simulink model "PIDPitch"  (R2012b)
settings: Solver=FixedStepDiscrete  StartTime=0.0  StopTime=9.96  FixedStep=Ts  RelTol=1e-3
values from neighbouring files (symbols this model uses):
  esc = esc+1    [bateria.m]
undefined symbols (not defined in the file or in its folder): DiscIntNeverNeededParam, Ts
libraries: simulink x2, slident x1
settings Model: Creator=TOSHIBA  LastModifiedBy=Carlos
settings ConfigurationSet: Description=SimMechanics 2G

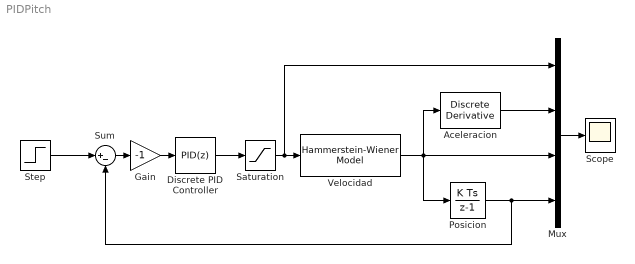
== system PIDPitch ==
  Aceleracion : simulink/Discrete/Discrete Derivative  gainval=1.0  ICPrevScaledInput=0.0  InputProcessing=Inherited  OutMin=[]  OutMax=[]  OutDataType=fixdt(1, 16)  OutScaling=2^-10  DoSatur=off
  Discrete PID Controller : simulink/Continuous/PID Controller  Controller=PID  TimeDomain=Discrete-time  SampleTime=Ts  IntegratorMethod=Forward Euler  FilterMethod=Forward Euler  Form=Parallel  P=0.7  I=0  D=0.5  N=15  InitialConditionSource=internal  InitialConditionForIntegrator=0  InitialConditionForFilter=0  ExternalReset=none  LimitOutput=off  UpperSaturationLimit=inf  LowerSaturationLimit=-inf  LinearizeAsGain=off  AntiWindupMode=none  Kb=1  TrackingMode=off  Kt=1  PParamMin=[]  PParamMax=[]  IParamMin=[]  IParamMax=[]  DParamMin=[]  DParamMax=[]  NParamMin=[]  NParamMax=[]  KbParamMin=[]  KbParamMax=[]  KtParamMin=[]  KtParamMax=[]  POutMin=[]  POutMax=[]  IOutMin=[]  IOutMax=[]  DOutMin=[]  DOutMax=[]  NOutMin=[]  NOutMax=[]  KbOutMin=[]  KbOutMax=[]  KtOutMin=[]  KtOutMax=[]  IntegratorOutMin=[]  IntegratorOutMax=[]  FilterOutMin=[]  FilterOutMax=[]  SumOutMin=[]  SumOutMax=[]  SumI1OutMin=[]  SumI1OutMax=[]  SumI2OutMin=[]  SumI2OutMax=[]  SumI3OutMin=[]  SumI3OutMax=[]  SumDOutMin=[]  SumDOutMax=[]  SaturationOutMin=[]  SaturationOutMax=[]  IntegratorContinuousStateAttributes=''  IntegratorStateMustResolveToSignalObject=off  IntegratorRTWStateStorageClass=Auto  FilterContinuousStateAttributes=''  FilterStateMustResolveToSignalObject=off  FilterRTWStateStorageClass=Auto
  Gain : Gain  Gain=-1  SampleTime=Ts
  Mux : Mux
  Posicion : DiscreteIntegrator  SampleTime=Ts  ICPrevOutput=DiscIntNeverNeededParam  ICPrevScaledInput=DiscIntNeverNeededParam
  Saturation : Saturate  UpperLimit=1  LowerLimit=-1  SampleTime=Ts
  Scope : Scope
      settings: SaveName=scdatavx  SampleInput=on  SampleTime=Ts
  Step : Step  After=esc  SampleTime=Ts
  Sum : Sum  Inputs=|+-  SampleTime=Ts
  Velocidad : slident/Hammerstein-Wiener Model  sys=vx123_nlhw113_pic2  IC=Zero  X0i=0
  wires:
  Velocidad/1 -> Aceleracion/1, Mux/3, Posicion/1
  Step/1 -> Sum/1
  Posicion/1 -> Sum/2, Mux/4
  Sum/1 -> Gain/1
  Gain/1 -> Discrete PID Controller/1
  Saturation/1 -> Mux/1, Velocidad/1
  Mux/1 -> Scope/1
  Discrete PID Controller/1 -> Saturation/1
  Aceleracion/1 -> Mux/2
